simulink model "diesel_prueba"  (R2018a)
settings: Solver=ode8  StartTime=0.0  StopTime=50  FixedStep=0.0001  RelTol=1e-3
InitFcn:
  | SimulinkInit_linea_transmision
values from neighbouring files (symbols this model uses):
  C3 = 610e-6    (= 0.00061)    [SimulinkInit_linea_transmision.m]
  Jd = 0.3    [SimulinkInit_linea_transmision.m]
  K1d = 1.15    [SimulinkInit_linea_transmision.m]
  K2d = 1    [SimulinkInit_linea_transmision.m]
  K3d = 1    [SimulinkInit_linea_transmision.m]
  L3 = 5e-3    (= 0.005)    [SimulinkInit_linea_transmision.m]
  L6 = 10e-6    (= 1e-05)    [SimulinkInit_linea_transmision.m]
  Pd = 0.1    [SimulinkInit_linea_transmision.m]
  R3 = 1e-3    (= 0.001)    [SimulinkInit_linea_transmision.m]
  R6 = 0.001    [SimulinkInit_linea_transmision.m]
  Tao1d = 0.5    [SimulinkInit_linea_transmision.m]
  Tao2d = 0.125    [SimulinkInit_linea_transmision.m]
libraries: simulink x1, powerlib_meascontrol x1
settings Model: Creator=MarioAndres  LastModifiedBy=cmparedes
settings OptimizationCC: DefaultParameterBehavior=Inlined  EnhancedBackFolding=on  PassReuseOutputArgsAs=Individual arguments  OptimizeBlockOrder=speed  DifferentSizesBufferReuse=on  OptimizationCustomize=off
settings DebuggingCC: ParameterTunabilityLossMsg=error
settings SFSimCC: MATLABDynamicMemAlloc=off
settings RTWCC: SystemTargetFile=ert.tlc  TemplateMakefile=ert_default_tmf  GenerateReport=on  IncludeHyperlinkInReport=on  LaunchReport=on  GenerateTraceInfo=on  GenerateTraceReport=on  GenerateTraceReportSl=on  GenerateTraceReportSf=on  GenerateTraceReportEml=on
settings CodeAppCC: ForceParamTrailComments=on  IgnoreCustomStorageClasses=off  OperatorAnnotations=on  SimulinkDataObjDesc=on  SFDataObjDesc=on  InsertBlockDesc=on
settings ERTTargetCC: TargetLangStandard=C99 (ISO)  GenerateSampleERTMain=on  SupportContinuousTime=on  InlinedParameterPlacement=NonHierarchical  ERTCustomFileTemplate=example_file_process.tlc

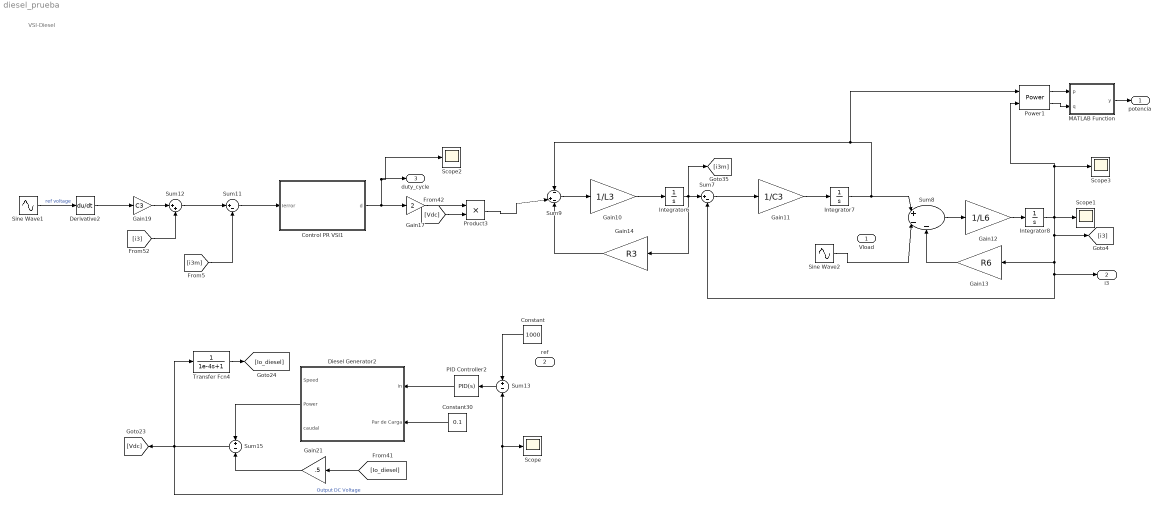
== system diesel_prueba ==
  note: VSI-Diesel
  "Vload " : Inport
  ref : Inport  Port=2
  Constant : Constant  Value=1000
  Constant30 : Constant  Value=0.1
  Control PR VSI1 : Subsystem
  Derivative2 : Derivative  CoefficientInTFapproximation=0
  Diesel Generator2 : Subsystem
  Gain10 : Gain  Gain=1/L3
  Gain11 : Gain  Gain=1/C3
  Gain12 : Gain  Gain=1/L6
  Gain13 : Gain  Gain=R6
  Gain14 : Gain  Gain=R3
  Gain17 : Gain  Gain=2
  Gain19 : Gain  Gain=C3
  Gain21 : Gain  Gain=.5
  Integrator6 : Integrator
  Integrator7 : Integrator
  Integrator8 : Integrator
  MATLAB Function : MATLAB Function  TreatAsAtomicUnit=on
  PID Controller2 : simulink/Continuous/PID Controller  Controller=PID  TimeDomain=Continuous-time  SampleTime=-1  IntegratorMethod=Forward Euler  FilterMethod=Forward Euler  Form=Parallel  UseFilter=on  ControllerParametersSource=internal  P=0.000853612192208084  I=3.94394231511782e-05  D=0.00224356290205903  N=0.155980576752107  InitialConditionSource=internal  InitialConditionForIntegrator=0  InitialConditionForFilter=0  ExternalReset=none  LimitOutput=off  UpperSaturationLimit=inf  LowerSaturationLimit=-inf  LinearizeAsGain=on  AntiWindupMode=none  Kb=1  TrackingMode=off  Kt=1  PParamMin=[]  PParamMax=[]  IParamMin=[]  IParamMax=[]  DParamMin=[]  DParamMax=[]  NParamMin=[]  NParamMax=[]  KbParamMin=[]  KbParamMax=[]  KtParamMin=[]  KtParamMax=[]  POutMin=[]  POutMax=[]  IOutMin=[]  IOutMax=[]  DOutMin=[]  DOutMax=[]  NOutMin=[]  NOutMax=[]  KbOutMin=[]  KbOutMax=[]  KtOutMin=[]  KtOutMax=[]  IntegratorOutMin=[]  IntegratorOutMax=[]  FilterOutMin=[]  FilterOutMax=[]  SumOutMin=[]  SumOutMax=[]  SumI1OutMin=[]  SumI1OutMax=[]  SumI2OutMin=[]  SumI2OutMax=[]  SumI3OutMin=[]  SumI3OutMax=[]  SumDOutMin=[]  SumDOutMax=[]  SaturationOutMin=[]  SaturationOutMax=[]  IntegratorContinuousStateAttributes=''  IntegratorStateMustResolveToSignalObject=off  IntegratorRTWStateStorageClass=Auto  FilterContinuousStateAttributes=''  FilterStateMustResolveToSignalObject=off  FilterRTWStateStorageClass=Auto  DifferentiatorICPrevScaledInput=0  DifferentiatorOutMin=[]  DifferentiatorOutMax=[]  InitialConditionSetting=State (most efficient)  FilterDiffOutCoefMin=[]  FilterDiffOutCoefMax=[]  SumDenOutMin=[]  SumDenOutMax=[]  SumNumOutMin=[]  SumNumOutMax=[]  ReciprocalOutMin=[]  ReciprocalOutMax=[]  DivideOutMin=[]  DivideOutMax=[]  TunerSelectOption=Transfer Function Based (PID Tuner App)
  Power1 : powerlib_meascontrol/Measurements/Power  Freq=60  Vinit=[1, 0]  Iinit=[1, 0]  Ts=0
      settings: SourceProductName=Simscape Power Systems
  Product3 : Product
  Scope{,1..3} (4 alike) : Scope
  Sine Wave1 : Sin  Amplitude=170  Frequency=2*pi*60  SampleTime=0
  Sine Wave2 : Sin  Amplitude=170  Frequency=2*pi*60  SampleTime=0
  Sum11 : Sum  Inputs=|+-
  Sum12 : Sum  Inputs=|++
  Sum13 : Sum  Inputs=+-
  Sum15 : Sum  Inputs=+-
  Sum7 : Sum  Inputs=|+-
  Sum8 : Sum  Inputs=|+--
  Sum9 : Sum  Inputs=-|+-
  Transfer Fcn4 : TransferFcn  Denominator=[1e-4 1]
  potencia : Outport
  i3 : Outport  Port=2
  duty_cycle : Outport  Port=3
  wires:
  Integrator7/1 -> Sum9/1, Power1/1, Sum8/1
  Sum12/1 -> Sum11/1
  Sum11/1 -> Control PR VSI1/1(Ierror)
  Gain19/1 -> Sum12/1
  Sum7/1 -> Gain11/1
  Gain12/1 -> Integrator8/1
  Integrator6/1 -> [i3m], Gain14/1, Sum7/1
  PID Controller2/1 -> Diesel Generator2/1(in)
  [i3m] -> Sum11/2
  Gain14/1 -> Sum9/3
  Gain11/1 -> Integrator7/1
  [Io_diesel] -> Gain21/1
  Sum8/1 -> Gain12/1
  Control PR VSI1/1(d) -> Scope2/1, duty_cycle/1, Gain17/1
  Diesel Generator2/2(Power) -> Sum15/1
  Gain21/1 -> Sum15/2
  Sum13/1 -> PID Controller2/1
  Transfer Fcn4/1 -> [Io_diesel]
  Constant30/1 -> Diesel Generator2/2(Par de Carga)
  Gain13/1 -> Sum8/3
  [Vdc] -> Product3/2
  [i3] -> Sum12/2
  Gain10/1 -> Integrator6/1
  Derivative2/1 -> Gain19/1
  Sum9/1 -> Gain10/1
  Gain17/1 -> Product3/1
  Sum15/1 -> [Vdc], Scope/1, Sum13/2, Transfer Fcn4/1  "Output DC Voltage"
  Sine Wave1/1 -> Derivative2/1  "ref voltage"
  Product3/1 -> Sum9/2
  Integrator8/1 -> Scope1/1, Scope3/1, Power1/2, [i3], Gain13/1, i3/1, Sum7/2
  Power1/1 -> MATLAB Function/1(p)
  Power1/2 -> MATLAB Function/2(q)
  MATLAB Function/1(y) -> potencia/1
  Constant/1 -> Sum13/1
  Sine Wave2/1 -> Sum8/2

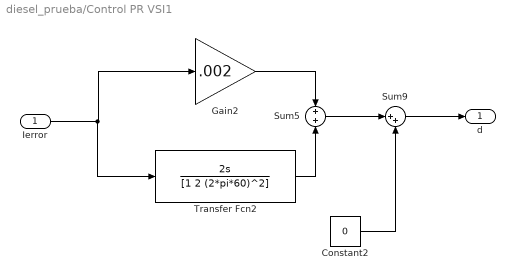
== system diesel_prueba/Control PR VSI1 ==
  Ierror : Inport
  Constant2 : Constant  Value=0
  Gain2 : Gain  Gain=.002
  Sum5 : Sum  Inputs=+|+
  Sum9 : Sum  Inputs=|++
  Transfer Fcn2 : TransferFcn  Numerator=[2 0]  Denominator=[1 2 (2*pi*60)^2]
  d : Outport
  wires:
  Constant2/1 -> Sum9/2
  Sum5/1 -> Sum9/1
  Transfer Fcn2/1 -> Sum5/2
  Gain2/1 -> Sum5/1
  Ierror/1 -> Transfer Fcn2/1, Gain2/1
  Sum9/1 -> d/1

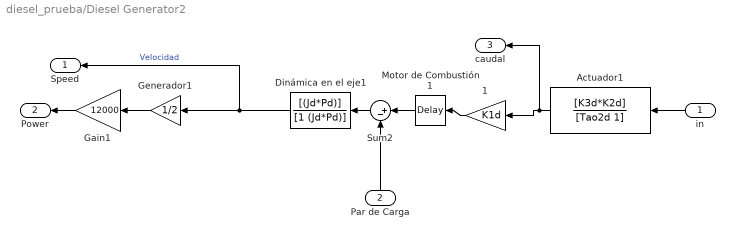
== system diesel_prueba/Diesel Generator2 ==
  in : Inport
  Par de Carga : Inport  Port=2
  " 1" : Gain  Gain=K1d
  " Generador1" : Gain  Gain=1/2
  Actuador1 : TransferFcn  Numerator=[K3d*K2d]  Denominator=[Tao2d 1]
  Dinámica en el eje1 : TransferFcn  Numerator=[(Jd*Pd)]  Denominator=[1 (Jd*Pd)]
  Gain1 : Gain  Gain=12000
  Motor de Combustión1 : TransportDelay  DelayTime=Tao1d
  Sum2 : Sum  Inputs=|+-
  Speed : Outport
  Power : Outport  Port=2
  caudal : Outport  Port=3
  wires:
  " 1"/1 -> Motor de Combustión1/1
  " Generador1"/1 -> Gain1/1
  Motor de Combustión1/1 -> Sum2/1
  Actuador1/1 -> caudal/1, " 1"/1
  Dinámica en el eje1/1 -> Speed/1, " Generador1"/1  "Velocidad"
  Sum2/1 -> Dinámica en el eje1/1
  in/1 -> Actuador1/1
  Par de Carga/1 -> Sum2/2
  Gain1/1 -> Power/1

== matlab function diesel_prueba/MATLAB Function ==
  data: p input; y output; q input
function y = fcn(p,q)

y = sqrt(p^2+q^2);
